simulink model "Controles11deJunio"  (R2022b)
settings: Solver=ode4  StartTime=0.0  StopTime=20  FixedStep=0.01  RelTol=1e-3
values from neighbouring files (symbols this model uses):
  A = [-1 -2 ... (first row only)    [ABinvariantes11deJunio.m]    (also in Convertibility.m = [0 1 0  0 0; DivirsoresElementales.m = [1 0 -1; 0 1 0; 0 0 2]; Examen.m = [1 1;0 1]; Examen2.m = [0 0  0 0 0)
  B = [1 ... (first row only)    [ABinvariantes11deJunio.m]    (also in Convertibility.m = [0 0; Examen.m = [1;0]; Examen2.m = [1 0; Sestrella.m = [0;1;0])
  D = [2 -3]    [ABinvariantes11deJunio.m]    (also in Examen2.m = [0 0 0 1 0]; V_estrella.m = [0 0 0 1 0]; Westrella.m = [1 0)
  K = place(A,B,P)    [ABinvariantes11deJunio.m]
  S = [3 ... (first row only)    [ABinvariantes11deJunio.m]    (also in Examen2.m = [1 0)
  Vd = yd/H0    (= -10)    [ABinvariantes11deJunio.m]
settings Model: Creator=raul  LastModifiedBy=raul

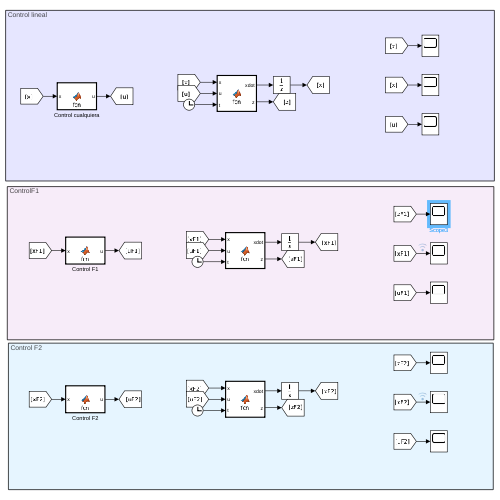
[thumbnail: Simulink's stored preview of the top-level diagram]
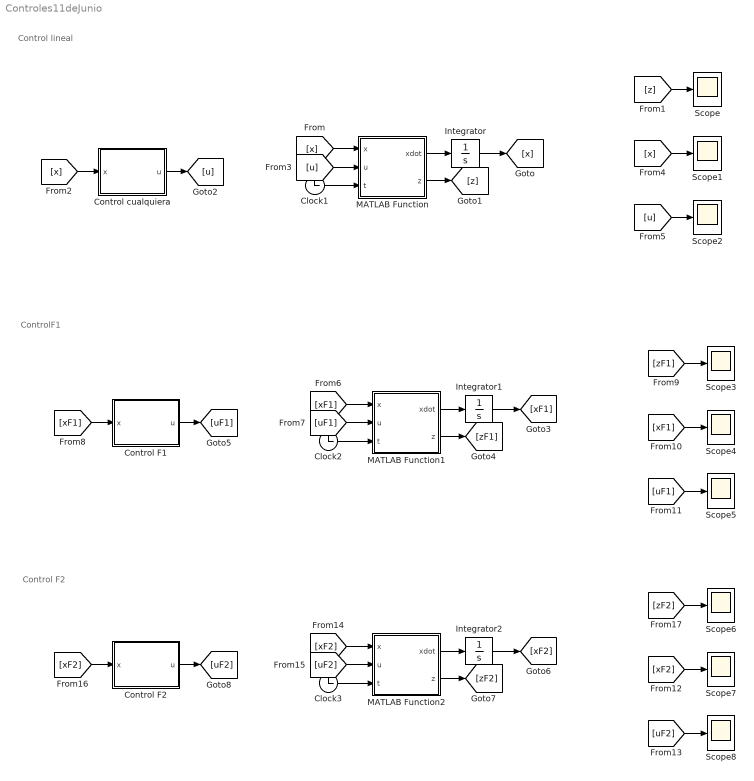
== system Controles11deJunio ==
  note: Control F2
  note: ControlF1
  note: Control lineal
  Clock1 : Clock
  Clock2 : Clock
  Clock3 : Clock
  Control F1 : MATLAB Function  TreatAsAtomicUnit=on
  Control F2 : MATLAB Function  TreatAsAtomicUnit=on
  Control cualquiera : MATLAB Function  TreatAsAtomicUnit=on
  Integrator : Integrator  InitialCondition=[0;0]
  Integrator1 : Integrator  InitialCondition=[1;2]
  Integrator2 : Integrator  InitialCondition=[5;3]
  MATLAB Function : MATLAB Function  TreatAsAtomicUnit=on
  MATLAB Function1 : MATLAB Function  TreatAsAtomicUnit=on
  MATLAB Function2 : MATLAB Function  TreatAsAtomicUnit=on
  Scope{,1..8} (9 alike) : Scope
  wires:
  MATLAB Function/1(xdot) -> Integrator/1
  Integrator/1 -> [x]
  [x] -> MATLAB Function/1(x)
  [z] -> Scope/1
  [x] -> Control cualquiera/1(x)
  [u] -> MATLAB Function/2(u)
  Control cualquiera/1(u) -> [u]
  Clock1/1 -> MATLAB Function/3(t)
  MATLAB Function/2(z) -> [z]
  [x] -> Scope1/1
  [u] -> Scope2/1
  Clock2/1 -> MATLAB Function1/3(t)
  MATLAB Function1/2(z) -> [zF1]
  [uF1] -> MATLAB Function1/2(u)
  Integrator1/1 -> [xF1]
  [xF1] -> MATLAB Function1/1(x)
  MATLAB Function1/1(xdot) -> Integrator1/1
  [xF1] -> Control F1/1(x)
  Control F1/1(u) -> [uF1]
  [uF1] -> Scope5/1
  [xF1] -> Scope4/1
  [zF1] -> Scope3/1
  [zF2] -> Scope6/1
  MATLAB Function2/2(z) -> [zF2]
  Clock3/1 -> MATLAB Function2/3(t)
  [uF2] -> MATLAB Function2/2(u)
  MATLAB Function2/1(xdot) -> Integrator2/1
  Integrator2/1 -> [xF2]
  [xF2] -> Control F2/1(x)
  [xF2] -> Scope7/1
  Control F2/1(u) -> [uF2]
  [xF2] -> MATLAB Function2/1(x)
  [uF2] -> Scope8/1

== matlab function Controles11deJunio/Control cualquiera ==
  data: u output; K parameter; x input; Vd parameter
function u = fcn(K,x, Vd)

u=-K*x+Vd;

== matlab function Controles11deJunio/MATLAB Function ==
  data: x input; A parameter; B parameter; u input; D parameter; S parameter; t input; xdot output; z output
function [xdot,z] = fcn(x, A, B, u, D, S,t)

if t<5
    q=0;
else
    q=cos(t);
end

xdot=A*x+B*u+S*q;

z = D*x;

== matlab function Controles11deJunio/MATLAB Function1 ==
  data: x input; A parameter; B parameter; u input; D parameter; S parameter; t input; xdot output; z output
function [xdot,z] = fcn(x, A, B, u, D, S,t)

if t<5
    q=0;
else
    q=cos(t);
end

xdot=A*x+B*u+S*q;

z = D*x;

== matlab function Controles11deJunio/Control F1 ==
  data: u output; Fp parameter; x input
function u = fcn(Fp,x)

u=Fp*x;

== matlab function Controles11deJunio/Control F2 ==
  data: u output; F2 parameter; x input
function u = fcn(F2,x)

u=F2*x;

== matlab function Controles11deJunio/MATLAB Function2 ==
  data: x input; A parameter; B parameter; u input; D parameter; S parameter; t input; xdot output; z output
function [xdot,z] = fcn(x, A, B, u, D, S,t)

if t<5
    q=0;
else
    q=cos(t);
end

xdot=A*x+B*u+S*q;

z = D*x;
